simulink model "obstacle_detector"  (R2016a)
settings: Solver=FixedStepAuto  StartTime=0.0  StopTime=inf  FixedStep=1  RelTol=1e-3
model workspace (MAT data in the model file):
  SL_ROS_VariableLengthArrays_MaxSizes.CommonInfo.ArrayTruncateAction = 'EmitWarning'
  SL_ROS_VariableLengthArrays_MaxSizes.MsgTypeMap = containers.Map
  SL_ROS_VariableLengthArrays_MaxSizes.MsgTypeMap.serialization.keys = {'sensor_msgs/LaserScan'}
  SL_ROS_VariableLengthArrays_MaxSizes.MsgTypeMap.serialization.values{1}(1).PropertyName = 'Ranges'
  SL_ROS_VariableLengthArrays_MaxSizes.MsgTypeMap.serialization.values{1}(1).DataType = 'single'
  SL_ROS_VariableLengthArrays_MaxSizes.MsgTypeMap.serialization.values{1}(1).MaxLength = 180
  SL_ROS_VariableLengthArrays_MaxSizes.MsgTypeMap.serialization.values{1}(2).PropertyName = 'Intensities'
  SL_ROS_VariableLengthArrays_MaxSizes.MsgTypeMap.serialization.values{1}(2).DataType = 'single'
  SL_ROS_VariableLengthArrays_MaxSizes.MsgTypeMap.serialization.values{1}(2).MaxLength = 180
  SL_ROS_VariableLengthArrays_MaxSizes.MsgTypeMap.serialization.uniformity = 0
  SL_ROS_VariableLengthArrays_MaxSizes.MsgTypeMap.serialization.keyType = 'char'
  SL_ROS_VariableLengthArrays_MaxSizes.MsgTypeMap.serialization.valueType = 'any'
undefined symbols (not defined in the file): Header
libraries: robotlib x4
settings Model: Creator=sprinkle  LastModifiedBy=ece446
settings OptimizationCC: OptimizeModelRefInitCode=on  LifeSpan=Inf  MaxStackSize=64
settings HardwareCC: ProdBitPerPointer=32  ProdLargestAtomicFloat=None  ProdIntDivRoundTo=Undefined  ProdEndianess=Unspecified  ProdWordSize=32  ProdHWDeviceType=Generic->Unspecified (assume 32-bit Generic)
settings RTWCC: SystemTargetFile=ert.tlc  HardwareBoard=Robot Operating System (ROS)  TemplateMakefile=ert_default_tmf  GenerateReport=on  Toolchain=Catkin  IncludeHyperlinkInReport=on  LaunchReport=on  TargetLang=C++  GenerateTraceInfo=on  GenerateTraceReport=on  GenerateTraceReportSl=on  GenerateTraceReportSf=on  GenerateTraceReportEml=on
settings CodeAppCC: ForceParamTrailComments=on  IgnoreCustomStorageClasses=off  OperatorAnnotations=on  SimulinkDataObjDesc=on  SFDataObjDesc=on  MATLABFcnDesc=on  InsertBlockDesc=on  MATLABSourceComments=on

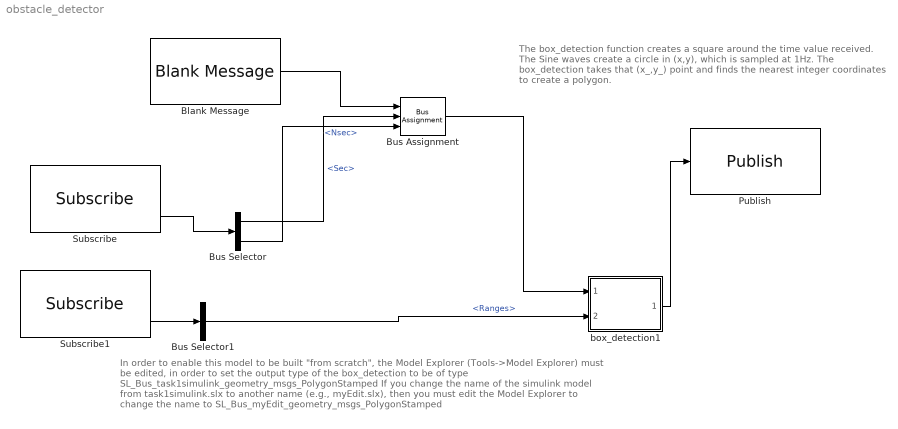
== system obstacle_detector ==
  note: In order to enable this model to be built "from scratch", the Model Explorer (Tools->Model Explorer) must be
      | edited, in order to set the output type of the box_detection to be of type
      | SL_Bus_task1simulink_geometry_msgs_PolygonStamped
      | If you change the name of the simulink model from task1simulink.slx to another name (e.g., myEdit.slx),
      | then you must edit the Model Explorer to change the name to
      | SL_Bus_myEdit_geometry_msgs_PolygonStamped
  note: The box_detection function creates a square around the time
      | value received. The Sine waves create a circle in (x,y), which
      | is sampled at 1Hz. The box_detection takes that (x_,y_) point
      | and finds the nearest integer coordinates to create a polygon.
  Blank Message : robotlib/Blank Message  SourceLibraryInfo=This block requires Robotics System Toolbox  messageType=geometry_msgs/PolygonStamped  SampleTime=inf
  Bus Assignment : BusAssignment  AssignedSignals=Header.Stamp.Sec,Header.Stamp.Nsec
  Bus Selector : BusSelector  OutputSignals=Clock_.Sec,Clock_.Nsec
  Bus Selector1 : BusSelector  OutputSignals=Ranges
  Publish : robotlib/Publish  SourceLibraryInfo=This block requires Robotics System Toolbox  topicSource=Specify your own  topic=/detections  messageType=geometry_msgs/PolygonStamped  messageQueueLength=1
  Subscribe : robotlib/Subscribe  SourceLibraryInfo=This block requires Robotics System Toolbox  topicSource=Select from ROS network  topic=/clock  messageType=rosgraph_msgs/Clock  sampleTime=-1  messageQueueLength=1
  Subscribe1 : robotlib/Subscribe  SourceLibraryInfo=This block requires Robotics System Toolbox  topicSource=Select from ROS network  topic=/catvehicle/front_laser_points  messageType=sensor_msgs/LaserScan  sampleTime=-1  messageQueueLength=1
  box_detection1 : MATLAB Function  TreatAsAtomicUnit=on
  wires:
  Blank Message/1 -> Bus Assignment/1
  Subscribe1/2 -> Bus Selector1/1
  Bus Assignment/1 -> box_detection1/1(blankMsg)
  box_detection1/1(outputMsg) -> Publish/1
  Bus Selector1/1 -> box_detection1/2(ranges)  "<Ranges>"
  Subscribe/2 -> Bus Selector/1
  Bus Selector/1 -> Bus Assignment/2  "<Sec>"
  Bus Selector/2 -> Bus Assignment/3  "<Nsec>"

== matlab function obstacle_detector/box_detection1 ==
  data: blankMsg input; ranges input; outputMsg output Bus: SL_Bus_obstacle_detector_geometry_msgs_PolygonStamped
    function outputMsg = fcn(blankMsg,ranges)
    %#codegen
    % the sequence of the message must increment each time we publish, so we
    % need it to be persistent across instantiations
    persistent seq;

    % if this is the first time our model is run, then 'seq' will not exist.
    % Then 'isempty(seq)' will be true, which allows us to intialize it to 0
    if isempty(seq)
        seq=uint32(0);
    end

    % increment the sequence number
    seq = seq+1;
    % set our output to be a copy of the input (blankMsg)
    outputMsg = blankMsg;

    % by definition in this block, we are making a square.
    % IF YOU USE THIS model as inspiration for an output detection that is a
    % pentagon, then you would set the length to be 5, for example.
    outputMsg.Polygon.Points_SL_Info.CurrentLength = uint32(4);
    % set the frame to be relative to our base of 0. If you want to use data
    % coming from another detection, then you can set the /detections to be in
    % the frame of that specific sensor
    str = 'catvehicle/odom';
    % initialize the header and set its values
    strLength = length(str);
    outputMsg.Header.Seq = seq;
    outputMsg.Header.FrameId(1:strLength) = str;
    outputMsg.Header.FrameId_SL_Info.CurrentLength = uint32(strLength);

    for idx=1:180
        if(ranges(idx)<80)
            % these points in (x,y,z) are either taken from the inputs, or hardcoded
            x = single(ranges(idx)*cosd(idx-90));
            y = single(ranges(idx)*sind(idx-90));
            z = single(0);
            % populate point 1
            outputMsg.Polygon.Points(1).X = floor(x);
            outputMsg.Polygon.Points(1).Y = floor(y);
            outputMsg.Polygon.Points(1).Z = z;
            
            % populate point 2
            outputMsg.Polygon.Points(2).X = floor(x);
            outputMsg.Polygon.Points(2).Y = ceil(y);
            outputMsg.Polygon.Points(2).Z = z;

            % populate point 3
            outputMsg.Polygon.Points(3).X = ceil(x);
            outputMsg.Polygon.Points(3).Y = ceil(y);
            outputMsg.Polygon.Points(3).Z = z;

            % populate point 4
            outputMsg.Polygon.Points(4).X = ceil(x);
            outputMsg.Polygon.Points(4).Y = floor(y);
            outputMsg.Polygon.Points(4).Z = z;
        end
    end

    % note that the polygon type "closes" between the last and first points


    % note that the polygon type "closes" between the last and first points
